simulink model "Drive_force_model"  (R2019b)
settings: Solver=VariableStepAuto  StartTime=0.0  StopTime=10.0  RelTol=1e-3
undefined symbols (not defined in the file or in its folder): Gear_ratio, Pedalling_force, torquefrommotor
settings Model: Creator=Avmash  LastModifiedBy=Avmash
settings DataIOCC: ReturnWorkspaceOutputs=off
settings DebuggingCC: ArithmeticOperatorsInVariantConditions=warning
settings SFSimCC: SimUseLocalCustomCode=off  CustomCodeUndefinedFunction=UseInterfaceOnly
settings RTWCC: RTWUseLocalCustomCode=off

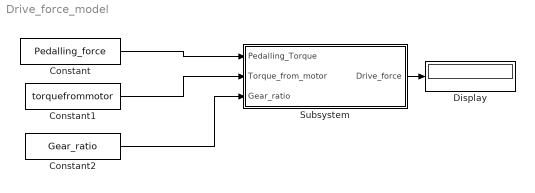
== system Drive_force_model ==
  Constant : Constant  Value=Pedalling_force
  Constant1 : Constant  Value=torquefrommotor
  Constant2 : Constant  Value=Gear_ratio
  Display : Display
  Subsystem : Subsystem
  wires:
  Constant1/1 -> Subsystem/2(Torque_from_motor)
  Constant/1 -> Subsystem/1(Pedalling_Torque)
  Subsystem/1(Drive_force) -> Display/1
  Constant2/1 -> Subsystem/3(Gear_ratio)

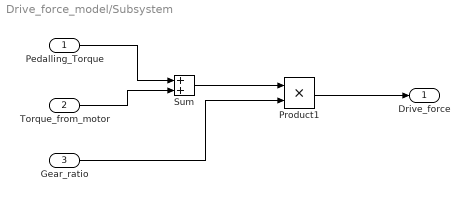
== system Drive_force_model/Subsystem ==
  Pedalling_Torque : Inport
  Torque_from_motor : Inport  Port=2
  Gear_ratio : Inport  Port=3
  Product1 : Product
  Sum : Sum
  Drive_force : Outport  VectorParamsAs1DForOutWhenUnconnected=off
  wires:
  Gear_ratio/1 -> Product1/2
  Product1/1 -> Drive_force/1
  Pedalling_Torque/1 -> Sum/1
  Torque_from_motor/1 -> Sum/2
  Sum/1 -> Product1/1
